simulink model "QPSK_synchronization_demo"  (R2021a)
settings: Solver=FixedStepDiscrete  StartTime=0.0  StopTime=inf  RelTol=1e-3
libraries: commfilt2 x2, commchan3 x1, commrandsrc3 x1, commdigbbndpm3 x1, simulink x1, commsync2 x1, dspsigops x1
settings Model: Creator=thomas  LastModifiedBy=student_1
settings SolverCC: AlgebraicLoopSolver=TrustRegion
settings DebuggingCC: SFMachineParentedDataDiag=warning

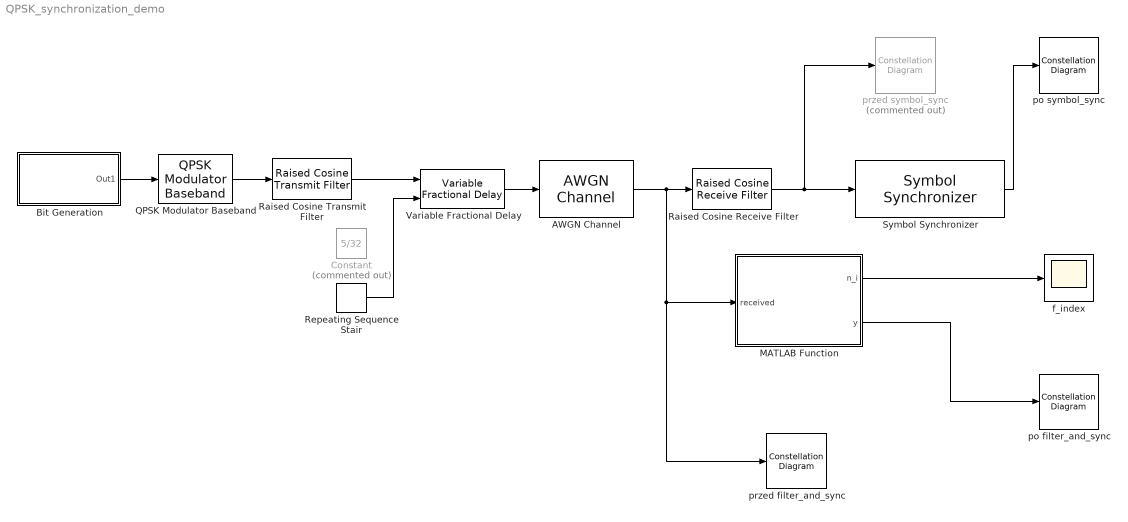
== system QPSK_synchronization_demo ==
  AWGN Channel : commchan3/AWGN Channel  InputProcessing=Columns as channels (frame based)  seed=67  noiseMode="Signal to noise ratio  (SNR)"  EbNodB=10  EsNodB=10  SNRdB=100  bitsPerSym=1  Ps=1/2  Tsym=1  variance=1
  Bit Generation : Subsystem
      mask Display: disp('Bit Frame\nGeneration')
  Constant : Constant  Commented=on  Value=5/32
  MATLAB Function : MATLAB Function  TreatAsAtomicUnit=on
  QPSK Modulator Baseband : commdigbbndpm3/QPSK Modulator Baseband  InType=Bit  Enc=Gray  Ph=pi/4  outDtype=double  outWordLen=16  outUDDataType=sfix(16)  outFracLenMode=Best precision  outFracLen=15  outDataTypeStr=double  outLastDataTypeStr=double
  Raised Cosine Receive Filter : commfilt2/Raised Cosine Receive Filter  filtType=Square root  R=0.2  filtSpan=10  N=2  downFactor=1  downOffset=0  filterGain=1  InputProcessing=Columns as channels (frame based)  RateOptions=Enforce single-rate processing  framing=Mute  checkCoeff=off  variableName=rcRxFilt  currentFiltSpan=10  D=5  inputOffset=0  sampMode=Mute  saveAsFlag=0  rateMode=Downsampling  checkGain=Normalized  launchFVT=on  roundingMode=Floor  overflowMode=off  coeffDataTypeStr=Inherit: Same word length as input  coeffMin=[]  coeffMax=[]  coeffLastDataTypeStr=Inherit: Same word length as input  accumDataTypeStr=Inherit: Same as product output  accumLastDataTypeStr=Inherit: Same as product output  outputDataTypeStr=Inherit: Same as accumulator  outputMin=[]  outputMax=[]  outputLastDataTypeStr=Inherit: Same as accumulator
  Raised Cosine Transmit Filter : commfilt2/Raised Cosine Transmit Filter  filtType=Square root  R=0.2  filtSpan=10  N=2  filterGain=1  InputProcessing=Columns as channels (frame based)  RateOptions=Enforce single-rate processing  framing=Mute  checkCoeff=off  variableName=rcTxFilt  checkGain=Normalized  sampMode=Mute  saveAsFlag=0  currentFiltSpan=10  D=(10)/2  launchFVT=on  roundingMode=Floor  overflowMode=off  coeffDataTypeStr=Inherit: Same word length as input  coeffMin=[]  coeffMax=[]  coeffLastDataTypeStr=Inherit: Same word length as input  outputDataTypeStr=Inherit: Same as accumulator  outputMin=[]  outputMax=[]  outputLastDataTypeStr=Inherit: Same as accumulator
  Repeating Sequence Stair : simulink/Sources/Repeating Sequence Stair  OutValues=[(1:1:31)/32 (31:-1:1)/32]  tsamp=-1  OutMin=[]  OutMax=[]  OutDataTypeStr=double  OutputDataTypeScalingMode=double  OutDataType=fixdt(0,8)  ConRadixGroup=Best Precision: Vector-wise  OutScaling=2^-12
  Symbol Synchronizer : commsync2/Symbol Synchronizer  Modulation=PAM/PSK/QAM  TimingErrorDetector=Zero-Crossing (decision-directed)  SamplesPerSymbol=2  DampingFactor=sqrt(2)/2  NormalizedLoopBandwidth=0.01  DetectorGain=2.7  TimingErrorOutputPort=off  SimulateUsing=Code generation
      settings: SourceProductBaseCode=CM
  Variable Fractional Delay : dspsigops/Variable Fractional Delay  mode=OBSOLETE  modeActive=Linear  L=4  FarrowL=4  R=10  alpha=1  dmax=400  InputProcessing=Columns as channels (frame based)  ic=0  noDFT=off  fallbackFIR=Clip to the minimum value necessary for centered kernel  fallbackFarrow=Clip to the minimum value necessary for centered kernel  roundingMode=Zero  overflowMode=off
      settings: SourceProductBaseCode=DS
  f_index : Scope
  po filter_and_sync : ConstellationDiagram
  po symbol_sync : ConstellationDiagram
  przed filter_and_sync : ConstellationDiagram
  przed symbol_sync : ConstellationDiagram  Commented=on
  wires:
  Raised Cosine Receive Filter/1 -> przed symbol_sync/1, Symbol Synchronizer/1
  Symbol Synchronizer/1 -> po symbol_sync/1
  Bit Generation/1(Out1) -> QPSK Modulator Baseband/1
  Raised Cosine Transmit Filter/1 -> Variable Fractional Delay/1
  QPSK Modulator Baseband/1 -> Raised Cosine Transmit Filter/1
  MATLAB Function/2(y) -> po filter_and_sync/1
  AWGN Channel/1 -> przed filter_and_sync/1, MATLAB Function/1(received), Raised Cosine Receive Filter/1
  Variable Fractional Delay/1 -> AWGN Channel/1
  MATLAB Function/1(n_i) -> f_index/1
  Repeating Sequence Stair/1 -> Variable Fractional Delay/2

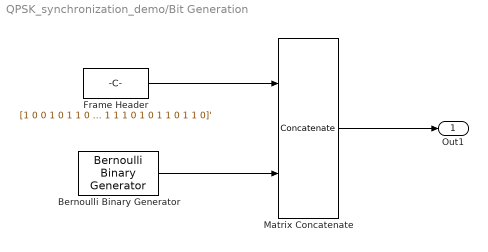
== system QPSK_synchronization_demo/Bit Generation ==
  Bernoulli Binary Generator : commrandsrc3/Bernoulli Binary Generator  ProbabilityOfZero=0.5  SeedSource=Parameter  Seed=61  SampleTime=1  SamplesPerFrame=160  OutputDataType=double  SimulateUsing=Interpreted execution
  Frame Header : Constant  Value=[1 0 0 1 0 1 1 0 1 1 1 0 1 0 1 1 0 1 1 0 1 0 0 1 0 1 1 0 1 1 1 0 1 0 1 1 0 1 1 0]'  VectorParams1D=off  OutDataTypeStr=double
  Matrix Concatenate : Concatenate  Mode=Multidimensional array
  Out1 : Outport  VectorParamsAs1DForOutWhenUnconnected=off
  wires:
  Matrix Concatenate/1 -> Out1/1
  Frame Header/1 -> Matrix Concatenate/1
  Bernoulli Binary Generator/1 -> Matrix Concatenate/2

== matlab function QPSK_synchronization_demo/MATLAB Function ==
  data: n_i output; y output size=300; received input
function [n_i, y] = filter_and_sync(received)

rolloff = 0.2;
symbols = 10;
sps = 64;
N2 = 32;
N1 = 2;
B = rcosdesign(rolloff, symbols,  sps, 'sqrt'); % odbiornik, filter enery is one
A = rcosdesign(rolloff, symbols,  N1, 'sqrt'); % odbiornik, filter enery is one
% B = B * N1;

rec_filtered = []; %zeros(32, length(received) + N1*symbols);
diff_rec_filtered = []; %zeros(32, length(received) + N1*symbols);

taps_per_filter = ceil(length(B)/N2);

B = [B, zeros(1, N2*taps_per_filter-length(B))];

difftaps = licz_diff(B, N2);
difftaps = [difftaps, zeros(1, N2*taps_per_filter-length(difftaps))];

for n=0:N2-1
   x = n : N2 : N2*taps_per_filter - 1;   

   skladowa_i = conv(real(received'), B(x+1),  'valid') ;
   skladowa_q = conv(imag(received'), B(x+1),  'valid') ;
   % przesuniecie o polowe dlugosci filtra
%    skladowa_i = skladowa_i(floor(taps_per_filter/2) + 1: end); 
%    skladowa_q = skladowa_q(floor(taps_per_filter/2) + 1: end); 
%    skladowa_i = skladowa_i(floor(length(received*N1)/2) + 1: end); 
%    skladowa_q = skladowa_q(floor(length(received*N1)/2) + 1: end);    

%    rec_filtered(n+1, : ) = skladowa_i + skladowa_q*1i;   
   rec_filtered = [rec_filtered; skladowa_i + skladowa_q*1i];

   diff_skladowa_i = conv(real(received'), difftaps(x+1), 'valid') ;
   diff_skladowa_q = conv(imag(received'), difftaps(x+1), 'valid')  ;
   % przesuniecie o polowe dlugosci filtra
%    diff_skladowa = diff_skladowa(floor(taps_per_filter/2) + 1: end);
%    diff_rec_filtered(n+1, : ) = diff_skladowa_i + diff_skladowa_q*1i;
   diff_rec_filtered = [diff_rec_filtered; diff_skladowa_i + diff_skladowa_q*1i]; 
   
end

two_rec_filtered = sqrt(sps/2)*rec_filtered( :, 1:2:end);
two_diff_rec_filtered = sqrt(sps/2)*diff_rec_filtered( :, 1:2:end);

% filter_indexes = [];
new_index = 1;  % obliczany indeks filtru z banków filtrów

% sprzężenie zwrotne - pętla PLL
CNT = 1;
CNT_next = 1;
underflow = 1;
vi = 0;

% na podstawie http://www.trondeau.com/blog/2011/8/13/control-loop-gain-values.html
Kp = 1.486;
damping_factor = 0.707;
loop_bw = 0.0628/4.69;

denom = Kp*(1 + 2*damping_factor*loop_bw + loop_bw*loop_bw);
K1= (4*damping_factor*loop_bw)/denom;
K2= (4*loop_bw*loop_bw)/denom;
 
% num_of_samples = length(received) + taps_per_filter - 1 - floor(taps_per_filter/2);
num_of_samples = length(received) - taps_per_filter + 1;
for n=1:num_of_samples
    CNT = CNT_next;
    if underflow == 1
        e = sign(real(rec_filtered(new_index, n))) * real(diff_rec_filtered(new_index, n));
%         e_q = sign(imag(rec_filtered(new_index, n))) * imag(diff_rec_filtered(new_index, n));
    else
        e = 0;
%         e_q = 0;
    end

%     e = sign(e)*sqrt(sqrt(abs(e)));
    % Loop filter - second order IIR
    vp = K1*e;
    vi = vi + K2*e;
    v = vp + vi;
    W = 1/2 + v;
%     vp_i = K1*e_i;
%     vi_i = vi_i + K2*e_i;
%     v_i = vp_i + vi_i;
%     W_i = 1/2 + v_i;

    CNT_next = CNT - W;

    if CNT_next < 0
        new_index = floor(rem(2*N2*abs(CNT_next), N2)) + 1;
%         filter_indexes = [filter_indexes, new_index];
        CNT_next = 1 + CNT_next;
        underflow = 1;
    else
        underflow = 0;
    end
end

% pamietac
y = two_rec_filtered(new_index, : )', n_i = new_index ;
